simulink model "Regelstrecke"  (R2025a)
settings: Solver=ode15s  StartTime=0.0  StopTime=10
model workspace (MATLAB code in the model file):
  | k = 1.380649e-23;
  | e = 1.602176634e-19;
  | T0 = 273.15;
  | 
  | IS = 1e-8;
  | R = 1e3;
  | L = 10e-3;
  | C1 = 100e-9;
  | C2 = 1e-6;
  | 
  | U0 = 12;
  | I0 = 6e-3;
  | 
  | G = [-0.9999 -1.1115 -995.9874; 0 -0.0005 -1];
settings Model: Creator=richa  LastModifiedBy=richa

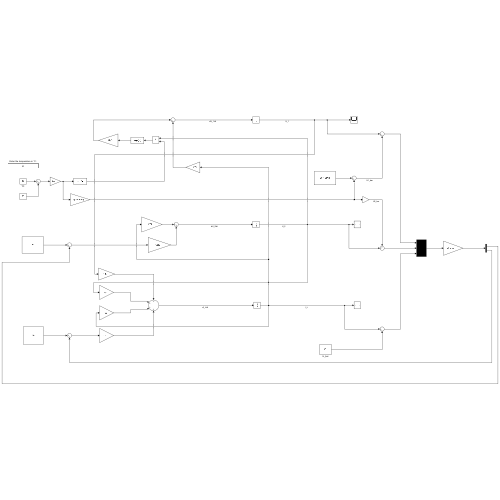
[thumbnail: Simulink's stored preview of the top-level diagram]
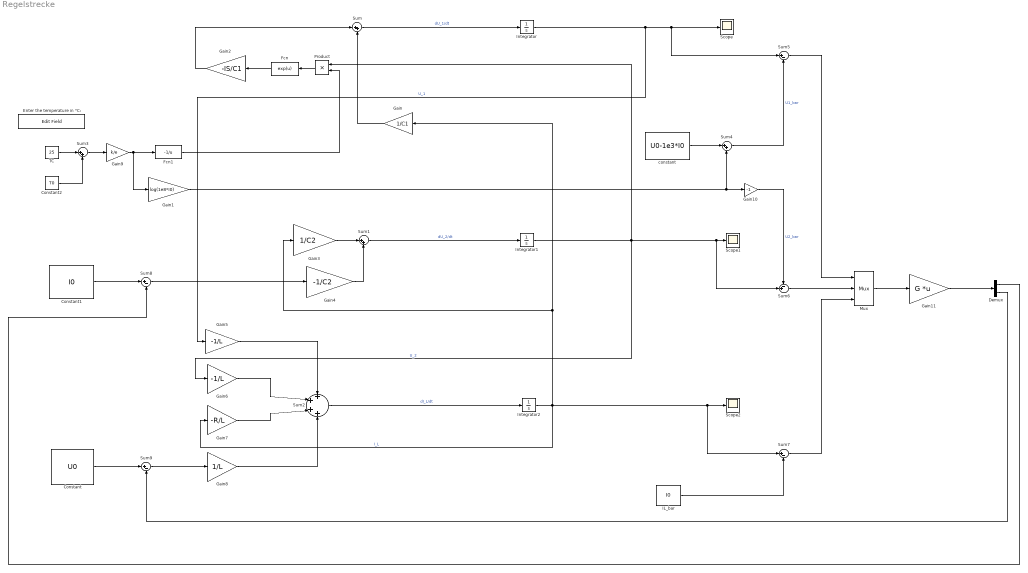
== system Regelstrecke ==
  Constant : Constant  Value=U0
  Constant1 : Constant  Value=I0
  Constant2 : Constant  Value=T0
  Demux : Demux  Outputs=2
  Enter the temperature in °C: : EditField  LabelPosition=Hide  ShowInitialText=on  Alignment=Center
  Fcn : Fcn  Expr=exp(u)
  Fcn1 : Fcn  Expr=-1/u
  Gain : Gain  Gain=1/C1
  Gain1 : Gain  Gain=log(1e8*I0)
  Gain10 : Gain  Gain=-1
  Gain11 : Gain  Gain=G  Multiplication=Matrix(K*u) (u vector)
  Gain2 : Gain  Gain=-IS/C1
  Gain3 : Gain  Gain=1/C2
  Gain4 : Gain  Gain=-1/C2
  Gain5 : Gain  Gain=-1/L
  Gain6 : Gain  Gain=-1/L
  Gain7 : Gain  Gain=-R/L
  Gain8 : Gain  Gain=1/L
  Gain9 : Gain  Gain=k/e
  IL_bar : Constant  Value=I0
  Integrator : Integrator
  Integrator1 : Integrator
  Integrator2 : Integrator
  Mux : Mux  Inputs=3
  Product : Product
  Scope : Scope
      settings: ActiveDisplayYMinimum=5.6640709824589885  ActiveDisplayYMaximum=7.426662358046614
  Scope1 : Scope
      settings: ActiveDisplayYMinimum=-0.35312832107088621  ActiveDisplayYMaximum=-0.27858609800218859
  Scope2 : Scope
      settings: ActiveDisplayYMinimum=0.0015441693561292953  ActiveDisplayYMaximum=0.0047644615133314193  DataLoggingVariableName=ScopeData2
  Sum{,1,3..4} (4 alike) : Sum  Inputs=|++
  Sum2 : Sum  Inputs=++++
  Sum{5,7..9} (4 alike) : Sum  Inputs=|+-
  Sum6 : Sum  Inputs=-+|
  TC : Constant  Value=25
  constant : Constant  Value=U0-1e3*I0
  wires:
  Integrator2/1 -> Sum7/1, Scope2/1, Gain7/1, Gain/1, Gain3/1  "I_L"
  Gain/1 -> Sum/2
  Integrator1/1 -> Sum6/2, Scope1/1, Product/1, Gain6/1  "U_2"
  Fcn/1 -> Gain2/1
  Gain2/1 -> Sum/1
  Sum/1 -> Integrator/1  "dU_1/dt"
  Gain3/1 -> Sum1/1
  Sum1/1 -> Integrator1/1  "dU_2/dt"
  Gain4/1 -> Sum1/2
  Integrator/1 -> Sum5/1, Scope/1, Gain5/1  "U_1"
  Gain5/1 -> Sum2/1
  Gain6/1 -> Sum2/2
  Gain7/1 -> Sum2/3
  Gain8/1 -> Sum2/4
  Sum2/1 -> Integrator2/1  "dI_L/dt"
  Gain9/1 -> Gain1/1, Fcn1/1
  Fcn1/1 -> Product/2
  Product/1 -> Fcn/1
  TC/1 -> Sum3/1
  Sum3/1 -> Gain9/1
  Constant2/1 -> Sum3/2
  constant/1 -> Sum4/1
  Gain1/1 -> Gain10/1, Sum4/2
  Sum4/1 -> Sum5/2  "U1_bar"
  Gain10/1 -> Sum6/1  "U2_bar"
  IL_bar/1 -> Sum7/2
  Mux/1 -> Gain11/1
  Gain11/1 -> Demux/1
  Sum6/1 -> Mux/2
  Sum5/1 -> Mux/1
  Sum7/1 -> Mux/3
  Constant1/1 -> Sum8/1
  Sum8/1 -> Gain4/1
  Constant/1 -> Sum9/1
  Sum9/1 -> Gain8/1
  Demux/2 -> Sum9/2
  Demux/1 -> Sum8/2
